simulink library "IO"  (R2024a)
settings: Solver=VariableStepAuto  StartTime=0.0  StopTime=10.0  RelTol=1e-3
values from neighbouring files (symbols this model uses):
  ADCBits = 12.0    [IO.sldd]
  Vref = 5.0    [IO.sldd]
undefined symbols (not defined in the file or in its folder): Bridge, dt, H, raptor_xcp_function
libraries: Raptor_lib x69, Utilities x20, Cooling x1
(part 3 of 3)

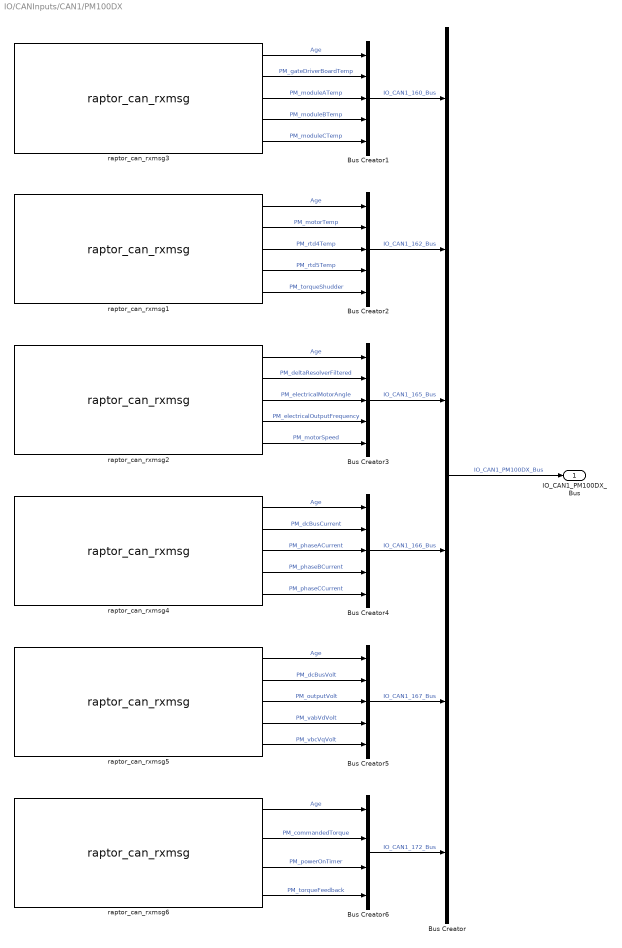
== system IO/CANInputs/CAN1/PM100DX ==
  Bus Creator : BusCreator  Inputs=6
  Bus Creator{1..5} (5 alike) : BusCreator  Inputs=5
  Bus Creator6 : BusCreator  Inputs=4
  raptor_can_rxmsg1 : Raptor_lib/CAN/raptor_can_rxmsg  canDefinition=struct('dbcFile', 'SR26_CAN1.dbc','message', 'PM_162','comment', '','signals', {{'PM_motorTemp','PM_rtd4Temp','PM_rtd5Temp','PM_torqueShudder'}},'enabled', [ 1 1 1 1;],'scaled', [ 1 1 1 1;],'canBus', '''CAN1''','messageID', [ 162;],'idMask', [ 536870911;],'payloadMask', [],'payloadValue', [],'period', [ 0;],'mailbox', '''''','queueSize', [ 1;],'label', [ 0;],'ver', [ 2;],'showID', [ 0;],'showRaw', [ 0;],'showRawMsg', [ 0;],'useStartVals', [ 0;],'extendedId', [ 0;],'showAge', [ 1;],'useSimFunc', [ 0;],'sim_func_name', '''''','fill', [ 0;],'editID', [ 0;],'signalOrder', [ 1;],'signalAscDes', [ 1;],'msgLength', [ 8;])  canBus='CAN1'  mailbox=''  payloadMask=[]  payloadValue=[]  idMask=hex2dec('1FFFFFFF')  queueSize=1  showID=0  label=0  fill=0  id=162  showRaw=0  showAge=1  signalOrder=1  signalInfo={{struct('Name', 'PM_torqueShudder','StartBit', [ 48;],'SignalSize', [ 16;],'ByteOrder', 'LittleEndian','ValueType', 'SIGNED','Class', 'int16','Signed', [ 1;],'Factor', [ 0.1;],'Offset', [ 0;],'Min', [ -3276.8;],'Max', [ 3276.7;],'Units', 'Nm','StartVal', [ 0;],'Comment', 'Shudder Compensation Value of Torque','Multiplexed', [ 0;],'Multiplexor', [ 0;],'MultiplexMode_Min', [],'MultiplexMode_Max', []),struct('Name', 'PM_motorTemp','StartBit', [ 32;],'SignalSize', [ 16;],'ByteOrder', 'LittleEndian','ValueType', 'SIGNED','Class', 'int16','Signed', [ 1;],'Factor', [ 0.1;],'Offset', [ 0;],'Min', [ -3276.8;],'Max', [ 3276.7;],'Units', 'degC','StartVal', [ 0;],'Comment', 'Motor Temperature Sensor','Multiplexed', [ 0;],'Multiplexor', [ 0;],'MultiplexMode_Min', [],'MultiplexMode_Max', []),struct('Name', 'PM_rtd5Temp','StartBit', [ 16;],'SignalSize', [ 16;],'ByteOrder', 'LittleEndian','ValueType', 'SIGNED','Class', 'int16','Signed', [ 1;],'Factor', [ 0.1;],'Offset', [ 0;],'Min', [ -3276.8;],'Max', [ 3276.7;],'Units', 'degC','StartVal', [ 0;],'Comment', 'RTD Input 5 (PT1000) Temperature (Gen 2 Only)','Multiplexed', [ 0;],'Multiplexor', [ 0;],'MultiplexMode_Min', [],'MultiplexMode_Max', []),struct('Name', 'PM_rtd4Temp','StartBit', [ 0;],'SignalSize', [ 16;],'ByteOrder', 'LittleEndian','ValueType', 'SIGNED','Class', 'int16','Signed', [ 1;],'Factor', [ 0.1;],'Offset', [ 0;],'Min', [ -3276.8;],'Max', [ 3276.7;],'Units', 'degC','StartVal', [ 0;],'Comment', 'RTD Input 4 (PT1000) Temperature (Gen 2 Only)','Multiplexed', [ 0;],'Multiplexor', [ 0;],'MultiplexMode_Min', [],'MultiplexMode_Max', [])}}  showRawMsg=0  useSimFunc=0  sim_func_name=''  useStartVals=0  extendedId=0
      settings: SourceProductName=Raptor
  raptor_can_rxmsg2 : Raptor_lib/CAN/raptor_can_rxmsg  canDefinition=struct('dbcFile', 'SR26_CAN1.dbc','message', 'PM_165','comment', '','signals', {{'PM_deltaResolverFiltered','PM_electricalMotorAngle','PM_electricalOutputFrequency','PM_motorSpeed'}},'enabled', [ 1 1 1 1;],'scaled', [ 1 1 1 1;],'canBus', '''CAN1''','messageID', [ 165;],'idMask', [ 536870911;],'payloadMask', [],'payloadValue', [],'period', [ 0;],'mailbox', '''''','queueSize', [ 1;],'label', [ 0;],'ver', [ 2;],'showID', [ 0;],'showRaw', [ 0;],'showRawMsg', [ 0;],'useStartVals', [ 0;],'extendedId', [ 0;],'showAge', [ 1;],'useSimFunc', [ 0;],'sim_func_name', '''''','fill', [ 0;],'editID', [ 0;],'signalOrder', [ 1;],'signalAscDes', [ 1;],'msgLength', [ 8;])  canBus='CAN1'  mailbox=''  payloadMask=[]  payloadValue=[]  idMask=hex2dec('1FFFFFFF')  queueSize=1  showID=0  label=0  fill=0  id=165  showRaw=0  showAge=1  signalOrder=1  signalInfo={{struct('Name', 'PM_deltaResolverFiltered','StartBit', [ 48;],'SignalSize', [ 16;],'ByteOrder', 'LittleEndian','ValueType', 'SIGNED','Class', 'int16','Signed', [ 1;],'Factor', [ 0.1;],'Offset', [ 0;],'Min', [ -3276.8;],'Max', [ 3276.7;],'Units', 'deg','StartVal', [ 0;],'Comment', 'Used in calibration of resolver angle adjustment','Multiplexed', [ 0;],'Multiplexor', [ 0;],'MultiplexMode_Min', [],'MultiplexMode_Max', []),struct('Name', 'PM_electricalOutputFrequency','StartBit', [ 32;],'SignalSize', [ 16;],'ByteOrder', 'LittleEndian','ValueType', 'SIGNED','Class', 'int16','Signed', [ 1;],'Factor', [ 0.1;],'Offset', [ 0;],'Min', [ -3276.8;],'Max', [ 3276.7;],'Units', 'Hz','StartVal', [ 0;],'Comment', 'The actual frequency of the inverter','Multiplexed', [ 0;],'Multiplexor', [ 0;],'MultiplexMode_Min', [],'MultiplexMode_Max', []),struct('Name', 'PM_motorSpeed','StartBit', [ 16;],'SignalSize', [ 16;],'ByteOrder', 'LittleEndian','ValueType', 'SIGNED','Class', 'int16','Signed', [ 1;],'Factor', [ 1;],'Offset', [ 0;],'Min', [ -32768;],'Max', [ 32767;],'Units', 'rpm','StartVal', [ 0;],'Comment', 'The measured speed of the motor','Multiplexed', [ 0;],'Multiplexor', [ 0;],'MultiplexMode_Min', [],'MultiplexMode_Max', []),struct('Name', 'PM_electricalMotorAngle','StartBit', [ 0;],'SignalSize', [ 16;],'ByteOrder', 'LittleEndian','ValueType', 'UNSIGNED','Class', 'uint16','Signed', [ 0;],'Factor', [ 0.1;],'Offset', [ 0;],'Min', [ 0;],'Max', [ 6553.5;],'Units', 'deg','StartVal', [ 0;],'Comment', 'The Electrical Angle of the motor as read by the encoder or resolver','Multiplexed', [ 0;],'Multiplexor', [ 0;],'MultiplexMode_Min', [],'MultiplexMode_Max', [])}}  showRawMsg=0  useSimFunc=0  sim_func_name=''  useStartVals=0  extendedId=0
      settings: SourceProductName=Raptor
  raptor_can_rxmsg3 : Raptor_lib/CAN/raptor_can_rxmsg  canDefinition=struct('dbcFile', 'SR26_CAN1.dbc','message', 'PM_160','comment', '','signals', {{'PM_gateDriverBoardTemp','PM_moduleATemp','PM_moduleBTemp','PM_moduleCTemp'}},'enabled', [ 1 1 1 1;],'scaled', [ 1 1 1 1;],'canBus', '''CAN1''','messageID', [ 160;],'idMask', [ 536870911;],'payloadMask', [],'payloadValue', [],'period', [ 0;],'mailbox', '''''','queueSize', [ 1;],'label', [ 0;],'ver', [ 2;],'showID', [ 0;],'showRaw', [ 0;],'showRawMsg', [ 0;],'useStartVals', [ 0;],'extendedId', [ 0;],'showAge', [ 1;],'useSimFunc', [ 0;],'sim_func_name', '''''','fill', [ 0;],'editID', [ 0;],'signalOrder', [ 1;],'signalAscDes', [ 1;],'msgLength', [ 8;])  canBus='CAN1'  mailbox=''  payloadMask=[]  payloadValue=[]  idMask=hex2dec('1FFFFFFF')  queueSize=1  showID=0  label=0  fill=0  id=160  showRaw=0  showAge=1  signalOrder=1  signalInfo={{struct('Name', 'PM_gateDriverBoardTemp','StartBit', [ 48;],'SignalSize', [ 16;],'ByteOrder', 'LittleEndian','ValueType', 'SIGNED','Class', 'int16','Signed', [ 1;],'Factor', [ 0.1;],'Offset', [ 0;],'Min', [ -3276.8;],'Max', [ 3276.7;],'Units', 'degC','StartVal', [ 0;],'Comment', 'Gate Driver Board Temperature','Multiplexed', [ 0;],'Multiplexor', [ 0;],'MultiplexMode_Min', [],'MultiplexMode_Max', []),struct('Name', 'PM_moduleCTemp','StartBit', [ 32;],'SignalSize', [ 16;],'ByteOrder', 'LittleEndian','ValueType', 'SIGNED','Class', 'int16','Signed', [ 1;],'Factor', [ 0.1;],'Offset', [ 0;],'Min', [ -3276.8;],'Max', [ 3276.7;],'Units', 'degC','StartVal', [ 0;],'Comment', 'IGBT Module C Temperature','Multiplexed', [ 0;],'Multiplexor', [ 0;],'MultiplexMode_Min', [],'MultiplexMode_Max', []),struct('Name', 'PM_moduleBTemp','StartBit', [ 16;],'SignalSize', [ 16;],'ByteOrder', 'LittleEndian','ValueType', 'SIGNED','Class', 'int16','Signed', [ 1;],'Factor', [ 0.1;],'Offset', [ 0;],'Min', [ -3276.8;],'Max', [ 3276.7;],'Units', 'degC','StartVal', [ 0;],'Comment', 'IGBT Module B Temperature','Multiplexed', [ 0;],'Multiplexor', [ 0;],'MultiplexMode_Min', [],'MultiplexMode_Max', []),struct('Name', 'PM_moduleATemp','StartBit', [ 0;],'SignalSize', [ 16;],'ByteOrder', 'LittleEndian','ValueType', 'SIGNED','Class', 'int16','Signed', [ 1;],'Factor', [ 0.1;],'Offset', [ 0;],'Min', [ -3276.8;],'Max', [ 3276.7;],'Units', 'degC','StartVal', [ 0;],'Comment', 'IGBT Module A Temperature','Multiplexed', [ 0;],'Multiplexor', [ 0;],'MultiplexMode_Min', [],'MultiplexMode_Max', [])}}  showRawMsg=0  useSimFunc=0  sim_func_name=''  useStartVals=0  extendedId=0
      settings: SourceProductName=Raptor
  raptor_can_rxmsg4 : Raptor_lib/CAN/raptor_can_rxmsg  canDefinition=struct('dbcFile', 'SR26_CAN1.dbc','message', 'PM_166','comment', '','signals', {{'PM_dcBusCurrent','PM_phaseACurrent','PM_phaseBCurrent','PM_phaseCCurrent'}},'enabled', [ 1 1 1 1;],'scaled', [ 1 1 1 1;],'canBus', '''CAN1''','messageID', [ 166;],'idMask', [ 536870911;],'payloadMask', [],'payloadValue', [],'period', [ 0;],'mailbox', '''''','queueSize', [ 1;],'label', [ 0;],'ver', [ 2;],'showID', [ 0;],'showRaw', [ 0;],'showRawMsg', [ 0;],'useStartVals', [ 0;],'extendedId', [ 0;],'showAge', [ 1;],'useSimFunc', [ 0;],'sim_func_name', '''''','fill', [ 0;],'editID', [ 0;],'signalOrder', [ 1;],'signalAscDes', [ 1;],'msgLength', [ 8;])  canBus='CAN1'  mailbox=''  payloadMask=[]  payloadValue=[]  idMask=hex2dec('1FFFFFFF')  queueSize=1  showID=0  label=0  fill=0  id=166  showRaw=0  showAge=1  signalOrder=1  signalInfo={{struct('Name', 'PM_dcBusCurrent','StartBit', [ 48;],'SignalSize', [ 16;],'ByteOrder', 'LittleEndian','ValueType', 'SIGNED','Class', 'int16','Signed', [ 1;],'Factor', [ 0.1;],'Offset', [ 0;],'Min', [ -3276.8;],'Max', [ 3276.7;],'Units', 'A','StartVal', [ 0;],'Comment', 'The calculated DC Bus Current','Multiplexed', [ 0;],'Multiplexor', [ 0;],'MultiplexMode_Min', [],'MultiplexMode_Max', []),struct('Name', 'PM_phaseCCurrent','StartBit', [ 32;],'SignalSize', [ 16;],'ByteOrder', 'LittleEndian','ValueType', 'SIGNED','Class', 'int16','Signed', [ 1;],'Factor', [ 0.1;],'Offset', [ 0;],'Min', [ -3276.8;],'Max', [ 3276.7;],'Units', 'A','StartVal', [ 0;],'Comment', 'The measured value of Phase C current','Multiplexed', [ 0;],'Multiplexor', [ 0;],'MultiplexMode_Min', [],'MultiplexMode_Max', []),struct('Name', 'PM_phaseBCurrent','StartBit', [ 16;],'SignalSize', [ 16;],'ByteOrder', 'LittleEndian','ValueType', 'SIGNED','Class', 'int16','Signed', [ 1;],'Factor', [ 0.1;],'Offset', [ 0;],'Min', [ -3276.8;],'Max', [ 3276.7;],'Units', 'A','StartVal', [ 0;],'Comment', 'The measured value of Phase B current','Multiplexed', [ 0;],'Multiplexor', [ 0;],'MultiplexMode_Min', [],'MultiplexMode_Max', []),struct('Name', 'PM_phaseACurrent','StartBit', [ 0;],'SignalSize', [ 16;],'ByteOrder', 'LittleEndian','ValueType', 'SIGNED','Class', 'int16','Signed', [ 1;],'Factor', [ 0.1;],'Offset', [ 0;],'Min', [ -3276.8;],'Max', [ 3276.7;],'Units', 'A','StartVal', [ 0;],'Comment', 'The measured value of Phase A current','Multiplexed', [ 0;],'Multiplexor', [ 0;],'MultiplexMode_Min', [],'MultiplexMode_Max', [])}}  showRawMsg=0  useSimFunc=0  sim_func_name=''  useStartVals=0  extendedId=0
      settings: SourceProductName=Raptor
  raptor_can_rxmsg5 : Raptor_lib/CAN/raptor_can_rxmsg  canDefinition=struct('dbcFile', 'SR26_CAN1.dbc','message', 'PM_167','comment', '','signals', {{'PM_dcBusVolt','PM_outputVolt','PM_vabVdVolt','PM_vbcVqVolt'}},'enabled', [ 1 1 1 1;],'scaled', [ 1 1 1 1;],'canBus', '''CAN1''','messageID', [ 167;],'idMask', [ 536870911;],'payloadMask', [],'payloadValue', [],'period', [ 0;],'mailbox', '''''','queueSize', [ 1;],'label', [ 0;],'ver', [ 2;],'showID', [ 0;],'showRaw', [ 0;],'showRawMsg', [ 0;],'useStartVals', [ 0;],'extendedId', [ 0;],'showAge', [ 1;],'useSimFunc', [ 0;],'sim_func_name', '''''','fill', [ 0;],'editID', [ 0;],'signalOrder', [ 1;],'signalAscDes', [ 1;],'msgLength', [ 8;])  canBus='CAN1'  mailbox=''  payloadMask=[]  payloadValue=[]  idMask=hex2dec('1FFFFFFF')  queueSize=1  showID=0  label=0  fill=0  id=167  showRaw=0  showAge=1  signalOrder=1  signalInfo={{struct('Name', 'PM_vbcVqVolt','StartBit', [ 48;],'SignalSize', [ 16;],'ByteOrder', 'LittleEndian','ValueType', 'SIGNED','Class', 'int16','Signed', [ 1;],'Factor', [ 0.1;],'Offset', [ 0;],'Min', [ -3276.8;],'Max', [ 3276.7;],'Units', 'V','StartVal', [ 0;],'Comment', 'Measured value of the voltage between Phase B and Phase C','Multiplexed', [ 0;],'Multiplexor', [ 0;],'MultiplexMode_Min', [],'MultiplexMode_Max', []),struct('Name', 'PM_vabVdVolt','StartBit', [ 32;],'SignalSize', [ 16;],'ByteOrder', 'LittleEndian','ValueType', 'SIGNED','Class', 'int16','Signed', [ 1;],'Factor', [ 0.1;],'Offset', [ 0;],'Min', [ -3276.8;],'Max', [ 3276.7;],'Units', 'V','StartVal', [ 0;],'Comment', 'Measured value of the voltage between Phase A and Phase B','Multiplexed', [ 0;],'Multiplexor', [ 0;],'MultiplexMode_Min', [],'MultiplexMode_Max', []),struct('Name', 'PM_outputVolt','StartBit', [ 16;],'SignalSize', [ 16;],'ByteOrder', 'LittleEndian','ValueType', 'SIGNED','Class', 'int16','Signed', [ 1;],'Factor', [ 0.1;],'Offset', [ 0;],'Min', [ -3276.8;],'Max', [ 3276.7;],'Units', 'V','StartVal', [ 0;],'Comment', 'The calculated value of the output voltage, in peak line-neutral volts','Multiplexed', [ 0;],'Multiplexor', [ 0;],'MultiplexMode_Min', [],'MultiplexMode_Max', []),struct('Name', 'PM_dcBusVolt','StartBit', [ 0;],'SignalSize', [ 16;],'ByteOrder', 'LittleEndian','ValueType', 'SIGNED','Class', 'int16','Signed', [ 1;],'Factor', [ 0.1;],'Offset', [ 0;],'Min', [ -3276.8;],'Max', [ 3276.7;],'Units', 'V','StartVal', [ 0;],'Comment', 'The actual measured value of the DC bus voltage','Multiplexed', [ 0;],'Multiplexor', [ 0;],'MultiplexMode_Min', [],'MultiplexMode_Max', [])}}  showRawMsg=0  useSimFunc=0  sim_func_name=''  useStartVals=0  extendedId=0
      settings: SourceProductName=Raptor
  raptor_can_rxmsg6 : Raptor_lib/CAN/raptor_can_rxmsg  canDefinition=struct('dbcFile', 'SR26_CAN1.dbc','message', 'PM_172','comment', '','signals', {{'PM_commandedTorque','PM_powerOnTimer','PM_torqueFeedback'}},'enabled', [ 1 1 1;],'scaled', [ 1 1 1;],'canBus', '''CAN1''','messageID', [ 172;],'idMask', [ 536870911;],'payloadMask', [],'payloadValue', [],'period', [ 0;],'mailbox', '''''','queueSize', [ 1;],'label', [ 0;],'ver', [ 2;],'showID', [ 0;],'showRaw', [ 0;],'showRawMsg', [ 0;],'useStartVals', [ 0;],'extendedId', [ 0;],'showAge', [ 1;],'useSimFunc', [ 0;],'sim_func_name', '''''','fill', [ 0;],'editID', [ 0;],'signalOrder', [ 1;],'signalAscDes', [ 1;],'msgLength', [ 8;])  canBus='CAN1'  mailbox=''  payloadMask=[]  payloadValue=[]  idMask=hex2dec('1FFFFFFF')  queueSize=1  showID=0  label=0  fill=0  id=172  showRaw=0  showAge=1  signalOrder=1  signalInfo={{struct('Name', 'PM_powerOnTimer','StartBit', [ 32;],'SignalSize', [ 32;],'ByteOrder', 'LittleEndian','ValueType', 'UNSIGNED','Class', 'uint32','Signed', [ 0;],'Factor', [ 0.003;],'Offset', [ 0;],'Min', [ 0;],'Max', [ 12884800;],'Units', 'sec','StartVal', [ 0;],'Comment', 'Updated every 3 msec. This will roll over in approximately 150 days!','Multiplexed', [ 0;],'Multiplexor', [ 0;],'MultiplexMode_Min', [],'MultiplexMode_Max', []),struct('Name', 'PM_torqueFeedback','StartBit', [ 16;],'SignalSize', [ 16;],'ByteOrder', 'LittleEndian','ValueType', 'SIGNED','Class', 'int16','Signed', [ 1;],'Factor', [ 0.1;],'Offset', [ 0;],'Min', [ -3276.8;],'Max', [ 3276.7;],'Units', 'Nm','StartVal', [ 0;],'Comment', 'Estimated motor torque feedback','Multiplexed', [ 0;],'Multiplexor', [ 0;],'MultiplexMode_Min', [],'MultiplexMode_Max', []),struct('Name', 'PM_commandedTorque','StartBit', [ 0;],'SignalSize', [ 16;],'ByteOrder', 'LittleEndian','ValueType', 'SIGNED','Class', 'int16','Signed', [ 1;],'Factor', [ 0.1;],'Offset', [ 0;],'Min', [ -3276.8;],'Max', [ 3276.7;],'Units', 'Nm','StartVal', [ 0;],'Comment', 'The commanded torque','Multiplexed', [ 0;],'Multiplexor', [ 0;],'MultiplexMode_Min', [],'MultiplexMode_Max', [])}}  showRawMsg=0  useSimFunc=0  sim_func_name=''  useStartVals=0  extendedId=0
      settings: SourceProductName=Raptor
  IO_CAN1_PM100DX_Bus : Outport
  wires:
  Bus Creator3/1 -> Bus Creator/3  "IO_CAN1_165_Bus"
  Bus Creator4/1 -> Bus Creator/4  "IO_CAN1_166_Bus"
  raptor_can_rxmsg6/4 -> Bus Creator6/4  "PM_torqueFeedback"
  raptor_can_rxmsg6/1 -> Bus Creator6/1  "Age"
  raptor_can_rxmsg6/2 -> Bus Creator6/2  "PM_commandedTorque"
  raptor_can_rxmsg6/3 -> Bus Creator6/3  "PM_powerOnTimer"
  Bus Creator6/1 -> Bus Creator/6  "IO_CAN1_172_Bus"
  Bus Creator5/1 -> Bus Creator/5  "IO_CAN1_167_Bus"
  raptor_can_rxmsg5/5 -> Bus Creator5/5  "PM_vbcVqVolt"
  raptor_can_rxmsg5/4 -> Bus Creator5/4  "PM_vabVdVolt"
  raptor_can_rxmsg5/3 -> Bus Creator5/3  "PM_outputVolt"
  raptor_can_rxmsg5/2 -> Bus Creator5/2  "PM_dcBusVolt"
  raptor_can_rxmsg5/1 -> Bus Creator5/1  "Age"
  raptor_can_rxmsg4/1 -> Bus Creator4/1  "Age"
  raptor_can_rxmsg4/2 -> Bus Creator4/2  "PM_dcBusCurrent"
  raptor_can_rxmsg4/3 -> Bus Creator4/3  "PM_phaseACurrent"
  raptor_can_rxmsg4/4 -> Bus Creator4/4  "PM_phaseBCurrent"
  raptor_can_rxmsg4/5 -> Bus Creator4/5  "PM_phaseCCurrent"
  raptor_can_rxmsg2/5 -> Bus Creator3/5  "PM_motorSpeed"
  raptor_can_rxmsg2/4 -> Bus Creator3/4  "PM_electricalOutputFrequency"
  raptor_can_rxmsg2/3 -> Bus Creator3/3  "PM_electricalMotorAngle"
  raptor_can_rxmsg2/2 -> Bus Creator3/2  "PM_deltaResolverFiltered"
  raptor_can_rxmsg2/1 -> Bus Creator3/1  "Age"
  raptor_can_rxmsg3/5 -> Bus Creator1/5  "PM_moduleCTemp"
  raptor_can_rxmsg3/4 -> Bus Creator1/4  "PM_moduleBTemp"
  raptor_can_rxmsg3/3 -> Bus Creator1/3  "PM_moduleATemp"
  raptor_can_rxmsg3/2 -> Bus Creator1/2  "PM_gateDriverBoardTemp"
  Bus Creator1/1 -> Bus Creator/1  "IO_CAN1_160_Bus"
  raptor_can_rxmsg3/1 -> Bus Creator1/1  "Age"
  Bus Creator/1 -> IO_CAN1_PM100DX_Bus/1  "IO_CAN1_PM100DX_Bus"
  raptor_can_rxmsg1/1 -> Bus Creator2/1  "Age"
  raptor_can_rxmsg1/2 -> Bus Creator2/2  "PM_motorTemp"
  raptor_can_rxmsg1/3 -> Bus Creator2/3  "PM_rtd4Temp"
  raptor_can_rxmsg1/4 -> Bus Creator2/4  "PM_rtd5Temp"
  raptor_can_rxmsg1/5 -> Bus Creator2/5  "PM_torqueShudder"
  Bus Creator2/1 -> Bus Creator/2  "IO_CAN1_162_Bus"

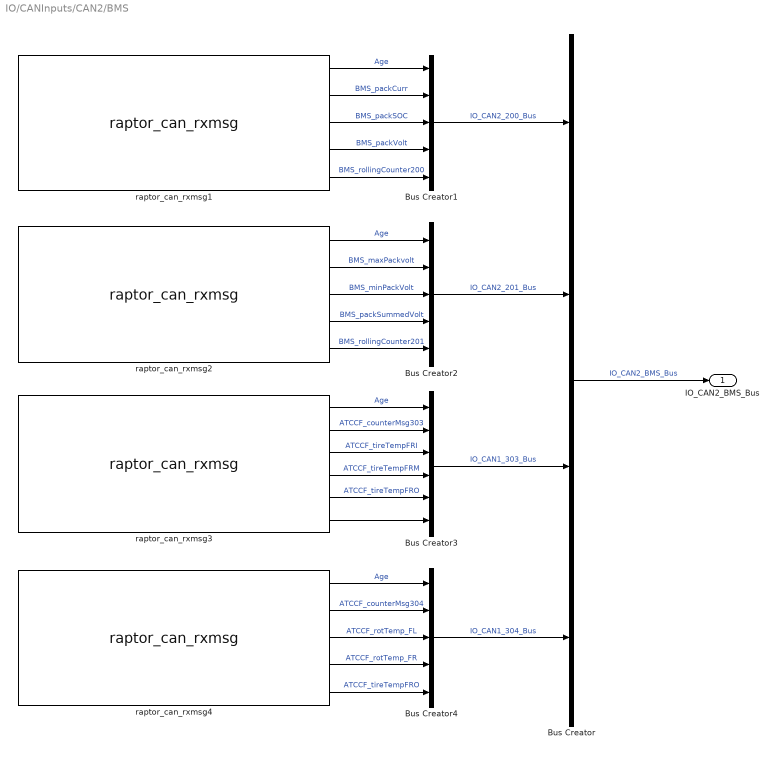
== system IO/CANInputs/CAN2/BMS ==
  Bus Creator : BusCreator  Inputs=4
  Bus Creator1 : BusCreator  Inputs=5
  Bus Creator2 : BusCreator  Inputs=5
  Bus Creator3 : BusCreator  Inputs=6
  Bus Creator4 : BusCreator  Inputs=5
  raptor_can_rxmsg1 : Raptor_lib/CAN/raptor_can_rxmsg  canDefinition=struct('dbcFile', 'SR26_CAN2.dbc','message', 'BMS_200','comment', '','signals', {{'BMS_packCurr','BMS_packSOC','BMS_packVolt','BMS_rollingCounter200'}},'enabled', [ 1 1 1 1;],'scaled', [ 1 1 1 1;],'canBus', '''CAN2''','messageID', [ 200;],'idMask', [ 536870911;],'payloadMask', [],'payloadValue', [],'period', [ 0;],'mailbox', '''''','queueSize', [ 1;],'label', [ 0;],'ver', [ 2;],'showID', [ 0;],'showRaw', [ 0;],'showRawMsg', [ 0;],'useStartVals', [ 0;],'extendedId', [ 0;],'showAge', [ 1;],'useSimFunc', [ 0;],'sim_func_name', '''''','fill', [ 0;],'editID', [ 0;],'signalOrder', [ 1;],'signalAscDes', [ 1;],'msgLength', [ 8;])  canBus='CAN2'  mailbox=''  payloadMask=[]  payloadValue=[]  idMask=hex2dec('1FFFFFFF')  queueSize=1  showID=0  label=0  fill=0  id=200  showRaw=0  showAge=1  signalOrder=1  signalInfo={{struct('Name', 'BMS_packSOC','StartBit', [ 48;],'SignalSize', [ 8;],'ByteOrder', 'LittleEndian','ValueType', 'SIGNED','Class', 'int8','Signed', [ 1;],'Factor', [ 0.5;],'Offset', [ 0;],'Min', [ 0;],'Max', [ 100;],'Units', '%','StartVal', [ 0;],'Comment', 'This is the pack State of Charge','Multiplexed', [ 0;],'Multiplexor', [ 0;],'MultiplexMode_Min', [],'MultiplexMode_Max', []),struct('Name', 'BMS_packVolt','StartBit', [ 32;],'SignalSize', [ 16;],'ByteOrder', 'LittleEndian','ValueType', 'SIGNED','Class', 'int16','Signed', [ 1;],'Factor', [ 0.1;],'Offset', [ 0;],'Min', [ -3276.8;],'Max', [ 3276.7;],'Units', 'V','StartVal', [ 0;],'Comment', 'This is the instantaneous total pack voltage value','Multiplexed', [ 0;],'Multiplexor', [ 0;],'MultiplexMode_Min', [],'MultiplexMode_Max', []),struct('Name', 'BMS_packCurr','StartBit', [ 16;],'SignalSize', [ 16;],'ByteOrder', 'LittleEndian','ValueType', 'SIGNED','Class', 'int16','Signed', [ 1;],'Factor', [ 0.1;],'Offset', [ 0;],'Min', [ -3276.8;],'Max', [ 3276.7;],'Units', 'A','StartVal', [ 0;],'Comment', 'This is the current pack amperage value for the battery pack. This will report a constant 0 if no current sensor is selected','Multiplexed', [ 0;],'Multiplexor', [ 0;],'MultiplexMode_Min', [],'MultiplexMode_Max', []),struct('Name', 'BMS_rollingCounter200','StartBit', [ 0;],'SignalSize', [ 8;],'ByteOrder', 'LittleEndian','ValueType', 'UNSIGNED','Class', 'uint8','Signed', [ 0;],'Factor', [ 1;],'Offset', [ 0;],'Min', [ 0;],'Max', [ 255;],'Units', '','StartVal', [ 0;],'Comment', 'Increments once every 100ms (max value is 255 and rolls over). Can be used to ensure data is updating','Multiplexed', [ 0;],'Multiplexor', [ 0;],'MultiplexMode_Min', [],'MultiplexMode_Max', [])}}  showRawMsg=0  useSimFunc=0  sim_func_name=''  useStartVals=0  extendedId=0
      settings: SourceProductName=Raptor
  raptor_can_rxmsg2 : Raptor_lib/CAN/raptor_can_rxmsg  canDefinition=struct('dbcFile', 'SR26_CAN2.dbc','message', 'BMS_201','comment', '','signals', {{'BMS_maxPackVolt','BMS_minPackVolt','BMS_packSummedVolt','BMS_rollingCounter201'}},'enabled', [ 1 1 1 1;],'scaled', [ 1 1 1 1;],'canBus', '''CAN2''','messageID', [ 201;],'idMask', [ 536870911;],'payloadMask', [],'payloadValue', [],'period', [ 0;],'mailbox', '''''','queueSize', [ 1;],'label', [ 0;],'ver', [ 2;],'showID', [ 0;],'showRaw', [ 0;],'showRawMsg', [ 0;],'useStartVals', [ 0;],'extendedId', [ 0;],'showAge', [ 1;],'useSimFunc', [ 0;],'sim_func_name', '''''','fill', [ 0;],'editID', [ 0;],'signalOrder', [ 1;],'signalAscDes', [ 1;],'msgLength', [ 8;])  canBus='CAN2'  mailbox=''  payloadMask=[]  payloadValue=[]  idMask=hex2dec('1FFFFFFF')  queueSize=1  showID=0  label=0  fill=0  id=201  showRaw=0  showAge=1  signalOrder=1  signalInfo={{struct('Name', 'BMS_minPackVolt','StartBit', [ 48;],'SignalSize', [ 16;],'ByteOrder', 'LittleEndian','ValueType', 'SIGNED','Class', 'int16','Signed', [ 1;],'Factor', [ 0.1;],'Offset', [ 0;],'Min', [ -3276.8;],'Max', [ 3276.7;],'Units', 'V','StartVal', [ 0;],'Comment', 'This value is the mainimum pack voltage that the BMS is using to limit how low the pack voltage is allowed to be pulled down to','Multiplexed', [ 0;],'Multiplexor', [ 0;],'MultiplexMode_Min', [],'MultiplexMode_Max', []),struct('Name', 'BMS_maxPackVolt','StartBit', [ 32;],'SignalSize', [ 16;],'ByteOrder', 'LittleEndian','ValueType', 'SIGNED','Class', 'int16','Signed', [ 1;],'Factor', [ 0.1;],'Offset', [ 0;],'Min', [ -3276.8;],'Max', [ 3276.7;],'Units', 'V','StartVal', [ 0;],'Comment', 'This value is the maximum pack voltage that the BMS is using to limit how high the pack voltage can be. This can be useful for communicating with chargers or charging stations expecting a maximum pack voltage value they are able to charge up to','Multiplexed', [ 0;],'Multiplexor', [ 0;],'MultiplexMode_Min', [],'MultiplexMode_Max', []),struct('Name', 'BMS_packSummedVolt','StartBit', [ 16;],'SignalSize', [ 16;],'ByteOrder', 'LittleEndian','ValueType', 'SIGNED','Class', 'int16','Signed', [ 1;],'Factor', [ 0.01;],'Offset', [ 0;],'Min', [ -327.68;],'Max', [ 327.67;],'Units', 'V','StartVal', [ 0;],'Comment', 'This value is the sum of all the cells being monitored by the BMS and represents the overall pack voltage. It is essentially identical to the Pack Voltage value, except that it is reported wit ha higher resolution (0.01V versus 0.1V)','Multiplexed', [ 0;],'Multiplexor', [ 0;],'MultiplexMode_Min', [],'MultiplexMode_Max', []),struct('Name', 'BMS_rollingCounter201','StartBit', [ 0;],'SignalSize', [ 8;],'ByteOrder', 'LittleEndian','ValueType', 'UNSIGNED','Class', 'uint8','Signed', [ 0;],'Factor', [ 1;],'Offset', [ 0;],'Min', [ 0;],'Max', [ 255;],'Units', '','StartVal', [ 0;],'Comment', 'Increments once every 100ms (max value is 255 and rolls over). Can be used to ensure data is updating','Multiplexed', [ 0;],'Multiplexor', [ 0;],'MultiplexMode_Min', [],'MultiplexMode_Max', [])}}  showRawMsg=0  useSimFunc=0  sim_func_name=''  useStartVals=0  extendedId=0
      settings: SourceProductName=Raptor
  raptor_can_rxmsg3 : Raptor_lib/CAN/raptor_can_rxmsg  canDefinition=struct('dbcFile', 'SR26_CAN2.dbc','message', 'BMS_202','comment', '','signals', {{'BMS_packAmphours','BMS_packDOD','BMS_packResistance','BMS_packSOH','BMS_rollingCounter202'}},'enabled', [ 1 1 1 1 1;],'scaled', [ 1 1 1 1 1;],'canBus', '''CAN2''','messageID', [ 202;],'idMask', [ 536870911;],'payloadMask', [],'payloadValue', [],'period', [ 0;],'mailbox', '''''','queueSize', [ 1;],'label', [ 0;],'ver', [ 2;],'showID', [ 0;],'showRaw', [ 0;],'showRawMsg', [ 0;],'useStartVals', [ 0;],'extendedId', [ 0;],'showAge', [ 1;],'useSimFunc', [ 0;],'sim_func_name', '''''','fill', [ 0;],'editID', [ 0;],'signalOrder', [ 1;],'signalAscDes', [ 1;],'msgLength', [ 8;])  canBus='CAN2'  mailbox=''  payloadMask=[]  payloadValue=[]  idMask=hex2dec('1FFFFFFF')  queueSize=1  showID=0  label=0  fill=0  id=202  showRaw=0  showAge=1  signalOrder=1  signalInfo={{struct('Name', 'BMS_packResistance','StartBit', [ 48;],'SignalSize', [ 16;],'ByteOrder', 'LittleEndian','ValueType', 'SIGNED','Class', 'int16','Signed', [ 1;],'Factor', [ 1;],'Offset', [ 0;],'Min', [ -32768;],'Max', [ 32767;],'Units', 'mOhm','StartVal', [ 0;],'Comment', 'This is the combined measured internal resistance for the entire battery pack','Multiplexed', [ 0;],'Multiplexor', [ 0;],'MultiplexMode_Min', [],'MultiplexMode_Max', []),struct('Name', 'BMS_packAmphours','StartBit', [ 32;],'SignalSize', [ 16;],'ByteOrder', 'LittleEndian','ValueType', 'SIGNED','Class', 'int16','Signed', [ 1;],'Factor', [ 0.1;],'Offset', [ 0;],'Min', [ -3276.8;],'Max', [ 3276.7;],'Units', 'Ahr','StartVal', [ 0;],'Comment', 'This is the calculated number of amphours remaining in the battery pack. This is used in part to calculate State of Charge','Multiplexed', [ 0;],'Multiplexor', [ 0;],'MultiplexMode_Min', [],'MultiplexMode_Max', []),struct('Name', 'BMS_packSOH','StartBit', [ 16;],'SignalSize', [ 8;],'ByteOrder', 'LittleEndian','ValueType', 'SIGNED','Class', 'int8','Signed', [ 1;],'Factor', [ 1;],'Offset', [ 0;],'Min', [ 0;],'Max', [ 100;],'Units', '%','StartVal', [ 0;],'Comment', 'This is the total state of health for the battery pack','Multiplexed', [ 0;],'Multiplexor', [ 0;],'MultiplexMode_Min', [],'MultiplexMode_Max', []),struct('Name', 'BMS_packDOD','StartBit', [ 8;],'SignalSize', [ 8;],'ByteOrder', 'LittleEndian','ValueType', 'SIGNED','Class', 'int8','Signed', [ 1;],'Factor', [ 0.5;],'Offset', [ 0;],'Min', [ 0;],'Max', [ 100;],'Units', '%','StartVal', [ 0;],'Comment', 'This value represents the total pack depth of discharge (that is, the total percent of the battery that has been discharged to this point). This value does not account for any Drift','Multiplexed', [ 0;],'Multiplexor', [ 0;],'MultiplexMode_Min', [],'MultiplexMode_Max', []),struct('Name', 'BMS_rollingCounter202','StartBit', [ 0;],'SignalSize', [ 8;],'ByteOrder', 'LittleEndian','ValueType', 'UNSIGNED','Class', 'uint8','Signed', [ 0;],'Factor', [ 1;],'Offset', [ 0;],'Min', [ 0;],'Max', [ 255;],'Units', '','StartVal', [ 0;],'Comment', 'Increments once every 100ms (max value is 255 and rolls over). Can be used to ensure data is updating','Multiplexed', [ 0;],'Multiplexor', [ 0;],'MultiplexMode_Min', [],'MultiplexMode_Max', [])}}  showRawMsg=0  useSimFunc=0  sim_func_name=''  useStartVals=0  extendedId=0
      settings: SourceProductName=Raptor
  raptor_can_rxmsg4 : Raptor_lib/CAN/raptor_can_rxmsg  canDefinition=struct('dbcFile', 'SR26_CAN2.dbc','message', 'BMS_201','comment', '','signals', {{'BMS_maxPackVolt','BMS_minPackVolt','BMS_packSummedVolt','BMS_rollingCounter201'}},'enabled', [ 1 1 1 1;],'scaled', [ 1 1 1 1;],'canBus', '''CAN2''','messageID', [ 201;],'idMask', [ 536870911;],'payloadMask', [],'payloadValue', [],'period', [ 0;],'mailbox', '''''','queueSize', [ 1;],'label', [ 0;],'ver', [ 2;],'showID', [ 0;],'showRaw', [ 0;],'showRawMsg', [ 0;],'useStartVals', [ 0;],'extendedId', [ 0;],'showAge', [ 1;],'useSimFunc', [ 0;],'sim_func_name', '''''','fill', [ 0;],'editID', [ 0;],'signalOrder', [ 1;],'signalAscDes', [ 1;],'msgLength', [ 8;])  canBus='CAN2'  mailbox=''  payloadMask=[]  payloadValue=[]  idMask=hex2dec('1FFFFFFF')  queueSize=1  showID=0  label=0  fill=0  id=201  showRaw=0  showAge=1  signalOrder=1  signalInfo={{struct('Name', 'BMS_minPackVolt','StartBit', [ 48;],'SignalSize', [ 16;],'ByteOrder', 'LittleEndian','ValueType', 'SIGNED','Class', 'int16','Signed', [ 1;],'Factor', [ 0.1;],'Offset', [ 0;],'Min', [ -3276.8;],'Max', [ 3276.7;],'Units', 'V','StartVal', [ 0;],'Comment', 'This value is the mainimum pack voltage that the BMS is using to limit how low the pack voltage is allowed to be pulled down to','Multiplexed', [ 0;],'Multiplexor', [ 0;],'MultiplexMode_Min', [],'MultiplexMode_Max', []),struct('Name', 'BMS_maxPackVolt','StartBit', [ 32;],'SignalSize', [ 16;],'ByteOrder', 'LittleEndian','ValueType', 'SIGNED','Class', 'int16','Signed', [ 1;],'Factor', [ 0.1;],'Offset', [ 0;],'Min', [ -3276.8;],'Max', [ 3276.7;],'Units', 'V','StartVal', [ 0;],'Comment', 'This value is the maximum pack voltage that the BMS is using to limit how high the pack voltage can be. This can be useful for communicating with chargers or charging stations expecting a maximum pack voltage value they are able to charge up to','Multiplexed', [ 0;],'Multiplexor', [ 0;],'MultiplexMode_Min', [],'MultiplexMode_Max', []),struct('Name', 'BMS_packSummedVolt','StartBit', [ 16;],'SignalSize', [ 16;],'ByteOrder', 'LittleEndian','ValueType', 'SIGNED','Class', 'int16','Signed', [ 1;],'Factor', [ 0.01;],'Offset', [ 0;],'Min', [ -327.68;],'Max', [ 327.67;],'Units', 'V','StartVal', [ 0;],'Comment', 'This value is the sum of all the cells being monitored by the BMS and represents the overall pack voltage. It is essentially identical to the Pack Voltage value, except that it is reported wit ha higher resolution (0.01V versus 0.1V)','Multiplexed', [ 0;],'Multiplexor', [ 0;],'MultiplexMode_Min', [],'MultiplexMode_Max', []),struct('Name', 'BMS_rollingCounter201','StartBit', [ 0;],'SignalSize', [ 8;],'ByteOrder', 'LittleEndian','ValueType', 'UNSIGNED','Class', 'uint8','Signed', [ 0;],'Factor', [ 1;],'Offset', [ 0;],'Min', [ 0;],'Max', [ 255;],'Units', '','StartVal', [ 0;],'Comment', 'Increments once every 100ms (max value is 255 and rolls over). Can be used to ensure data is updating','Multiplexed', [ 0;],'Multiplexor', [ 0;],'MultiplexMode_Min', [],'MultiplexMode_Max', [])}}  showRawMsg=0  useSimFunc=0  sim_func_name=''  useStartVals=0  extendedId=0
      settings: SourceProductName=Raptor
  IO_CAN2_BMS_Bus : Outport
  wires:
  raptor_can_rxmsg3/6 -> Bus Creator3/6
  raptor_can_rxmsg4/5 -> Bus Creator4/5  "ATCCF_tireTempFRO"
  raptor_can_rxmsg1/5 -> Bus Creator1/5  "BMS_rollingCounter200"
  Bus Creator1/1 -> Bus Creator/1  "IO_CAN2_200_Bus"
  raptor_can_rxmsg1/4 -> Bus Creator1/4  "BMS_packVolt"
  raptor_can_rxmsg1/3 -> Bus Creator1/3  "BMS_packSOC"
  raptor_can_rxmsg1/2 -> Bus Creator1/2  "BMS_packCurr"
  raptor_can_rxmsg1/1 -> Bus Creator1/1  "Age"
  raptor_can_rxmsg2/1 -> Bus Creator2/1  "Age"
  raptor_can_rxmsg2/2 -> Bus Creator2/2  "BMS_maxPackvolt"
  raptor_can_rxmsg2/3 -> Bus Creator2/3  "BMS_minPackVolt"
  raptor_can_rxmsg2/4 -> Bus Creator2/4  "BMS_packSummedVolt"
  Bus Creator2/1 -> Bus Creator/2  "IO_CAN2_201_Bus"
  raptor_can_rxmsg2/5 -> Bus Creator2/5  "BMS_rollingCounter201"
  raptor_can_rxmsg3/5 -> Bus Creator3/5  "ATCCF_tireTempFRO"
  Bus Creator3/1 -> Bus Creator/3  "IO_CAN1_303_Bus"
  raptor_can_rxmsg3/4 -> Bus Creator3/4  "ATCCF_tireTempFRM"
  raptor_can_rxmsg3/3 -> Bus Creator3/3  "ATCCF_tireTempFRI"
  raptor_can_rxmsg3/2 -> Bus Creator3/2  "ATCCF_counterMsg303"
  raptor_can_rxmsg3/1 -> Bus Creator3/1  "Age"
  raptor_can_rxmsg4/1 -> Bus Creator4/1  "Age"
  raptor_can_rxmsg4/2 -> Bus Creator4/2  "ATCCF_counterMsg304"
  raptor_can_rxmsg4/3 -> Bus Creator4/3  "ATCCF_rotTemp_FL"
  raptor_can_rxmsg4/4 -> Bus Creator4/4  "ATCCF_rotTemp_FR"
  Bus Creator4/1 -> Bus Creator/4  "IO_CAN1_304_Bus"
  Bus Creator/1 -> IO_CAN2_BMS_Bus/1  "IO_CAN2_BMS_Bus"

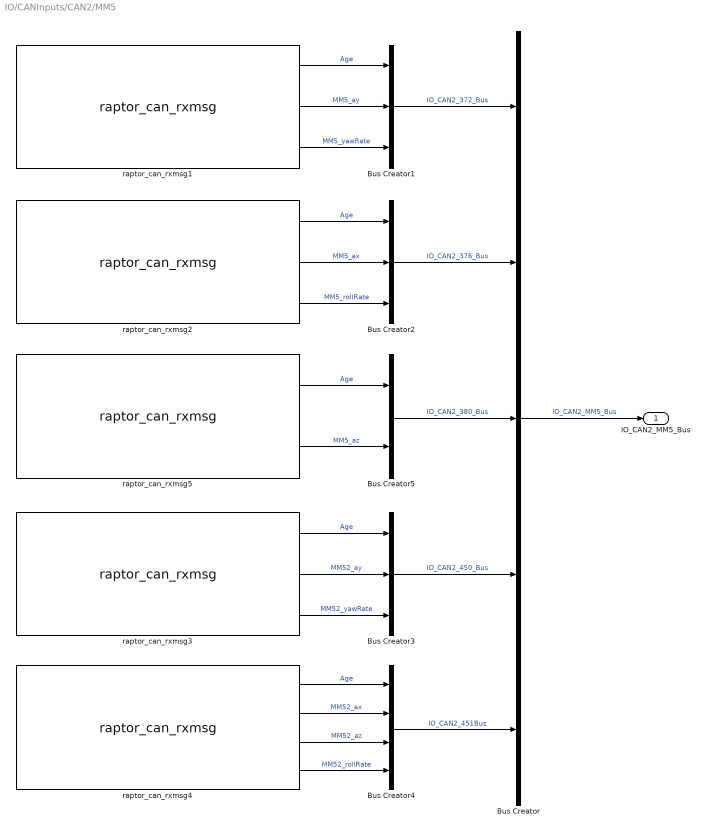
== system IO/CANInputs/CAN2/MM5 ==
  Bus Creator : BusCreator  Inputs=5
  Bus Creator1 : BusCreator  Inputs=3
  Bus Creator2 : BusCreator  Inputs=3
  Bus Creator3 : BusCreator  Inputs=3
  Bus Creator4 : BusCreator  Inputs=4
  Bus Creator5 : BusCreator  Inputs=2
  raptor_can_rxmsg1 : Raptor_lib/CAN/raptor_can_rxmsg  canDefinition=struct('dbcFile', 'SR26_CAN2.dbc','message', 'MM5_372','comment', '','signals', {{'MM5_ay','MM5_yawRate'}},'enabled', [ 1 1;],'scaled', [ 1 1;],'canBus', '''CAN2''','messageID', [ 372;],'idMask', [ 536870911;],'payloadMask', [],'payloadValue', [],'period', [ 0;],'mailbox', '''''','queueSize', [ 1;],'label', [ 0;],'ver', [ 2;],'showID', [ 0;],'showRaw', [ 0;],'showRawMsg', [ 0;],'useStartVals', [ 0;],'extendedId', [ 0;],'showAge', [ 1;],'useSimFunc', [ 0;],'sim_func_name', '''''','fill', [ 0;],'editID', [ 0;],'signalOrder', [ 1;],'signalAscDes', [ 1;],'msgLength', [ 8;])  canBus='CAN2'  mailbox=''  payloadMask=[]  payloadValue=[]  idMask=hex2dec('1FFFFFFF')  queueSize=1  showID=0  label=0  fill=0  id=372  showRaw=0  showAge=1  signalOrder=1  signalInfo={{struct('Name', 'MM5_ay','StartBit', [ 32;],'SignalSize', [ 16;],'ByteOrder', 'LittleEndian','ValueType', 'UNSIGNED','Class', 'uint16','Signed', [ 0;],'Factor', [ 0.0001274;],'Offset', [ -4.1746;],'Min', [ 0;],'Max', [ 0;],'Units', 'g','StartVal', [ 0;],'Comment', 'Acceleration Y Axis','Multiplexed', [ 0;],'Multiplexor', [ 0;],'MultiplexMode_Min', [],'MultiplexMode_Max', []),struct('Name', 'MM5_yawRate','StartBit', [ 0;],'SignalSize', [ 16;],'ByteOrder', 'LittleEndian','ValueType', 'UNSIGNED','Class', 'uint16','Signed', [ 0;],'Factor', [ 0.005;],'Offset', [ -163.9;],'Min', [ 0;],'Max', [ 0;],'Units', 'deg/sec','StartVal', [ 0;],'Comment', 'Yaw Rate','Multiplexed', [ 0;],'Multiplexor', [ 0;],'MultiplexMode_Min', [],'MultiplexMode_Max', [])}}  showRawMsg=0  useSimFunc=0  sim_func_name=''  useStartVals=0  extendedId=0
      settings: SourceProductName=Raptor
  raptor_can_rxmsg2 : Raptor_lib/CAN/raptor_can_rxmsg  canDefinition=struct('dbcFile', 'SR26_CAN2.dbc','message', 'MM5_376','comment', '','signals', {{'MM5_ax','MM5_rollRate'}},'enabled', [ 1 1;],'scaled', [ 1 1;],'canBus', '''CAN2''','messageID', [ 376;],'idMask', [ 536870911;],'payloadMask', [],'payloadValue', [],'period', [ 0;],'mailbox', '''''','queueSize', [ 1;],'label', [ 0;],'ver', [ 2;],'showID', [ 0;],'showRaw', [ 0;],'showRawMsg', [ 0;],'useStartVals', [ 0;],'extendedId', [ 0;],'showAge', [ 1;],'useSimFunc', [ 0;],'sim_func_name', '''''','fill', [ 0;],'editID', [ 0;],'signalOrder', [ 1;],'signalAscDes', [ 1;],'msgLength', [ 8;])  canBus='CAN2'  mailbox=''  payloadMask=[]  payloadValue=[]  idMask=hex2dec('1FFFFFFF')  queueSize=1  showID=0  label=0  fill=0  id=376  showRaw=0  showAge=1  signalOrder=1  signalInfo={{struct('Name', 'MM5_ax','StartBit', [ 32;],'SignalSize', [ 16;],'ByteOrder', 'LittleEndian','ValueType', 'UNSIGNED','Class', 'uint16','Signed', [ 0;],'Factor', [ -0.0001274;],'Offset', [ 4.1746;],'Min', [ 0;],'Max', [ 0;],'Units', 'g','StartVal', [ 0;],'Comment', 'Acceleration X Axis','Multiplexed', [ 0;],'Multiplexor', [ 0;],'MultiplexMode_Min', [],'MultiplexMode_Max', []),struct('Name', 'MM5_rollRate','StartBit', [ 0;],'SignalSize', [ 16;],'ByteOrder', 'LittleEndian','ValueType', 'UNSIGNED','Class', 'uint16','Signed', [ 0;],'Factor', [ -0.005;],'Offset', [ 163.9;],'Min', [ 0;],'Max', [ 0;],'Units', 'deg/sec','StartVal', [ 0;],'Comment', 'Roll Rate','Multiplexed', [ 0;],'Multiplexor', [ 0;],'MultiplexMode_Min', [],'MultiplexMode_Max', [])}}  showRawMsg=0  useSimFunc=0  sim_func_name=''  useStartVals=0  extendedId=0
      settings: SourceProductName=Raptor
  raptor_can_rxmsg3 : Raptor_lib/CAN/raptor_can_rxmsg  canDefinition=struct('dbcFile', 'SR26_CAN2.dbc','message', 'MM52_450','comment', '','signals', {{'MM52_ay','MM52_yawRate'}},'enabled', [ 1 1;],'scaled', [ 1 1;],'canBus', '''CAN2''','messageID', [ 450;],'idMask', [ 536870911;],'payloadMask', [],'payloadValue', [],'period', [ 0;],'mailbox', '''''','queueSize', [ 1;],'label', [ 0;],'ver', [ 2;],'showID', [ 0;],'showRaw', [ 0;],'showRawMsg', [ 0;],'useStartVals', [ 0;],'extendedId', [ 0;],'showAge', [ 1;],'useSimFunc', [ 0;],'sim_func_name', '''''','fill', [ 0;],'editID', [ 0;],'signalOrder', [ 1;],'signalAscDes', [ 1;],'msgLength', [ 8;])  canBus='CAN2'  mailbox=''  payloadMask=[]  payloadValue=[]  idMask=hex2dec('1FFFFFFF')  queueSize=1  showID=0  label=0  fill=0  id=450  showRaw=0  showAge=1  signalOrder=1  signalInfo={{struct('Name', 'MM52_ay','StartBit', [ 32;],'SignalSize', [ 16;],'ByteOrder', 'LittleEndian','ValueType', 'UNSIGNED','Class', 'uint16','Signed', [ 0;],'Factor', [ 0.0001274;],'Offset', [ -4.1746;],'Min', [ 0;],'Max', [ 0;],'Units', 'g','StartVal', [ 0;],'Comment', 'Acceleration Y Axis','Multiplexed', [ 0;],'Multiplexor', [ 0;],'MultiplexMode_Min', [],'MultiplexMode_Max', []),struct('Name', 'MM52_yawRate','StartBit', [ 0;],'SignalSize', [ 16;],'ByteOrder', 'LittleEndian','ValueType', 'UNSIGNED','Class', 'uint16','Signed', [ 0;],'Factor', [ 0.005;],'Offset', [ -163.9;],'Min', [ 0;],'Max', [ 0;],'Units', 'deg/sec','StartVal', [ 0;],'Comment', 'Yaw Rate','Multiplexed', [ 0;],'Multiplexor', [ 0;],'MultiplexMode_Min', [],'MultiplexMode_Max', [])}}  showRawMsg=0  useSimFunc=0  sim_func_name=''  useStartVals=0  extendedId=0
      settings: SourceProductName=Raptor
  raptor_can_rxmsg4 : Raptor_lib/CAN/raptor_can_rxmsg  canDefinition=struct('dbcFile', 'SR26_CAN2.dbc','message', 'MM52_451','comment', '','signals', {{'MM52_ax','MM52_az','MM52_rollRate'}},'enabled', [ 1 1 1;],'scaled', [ 1 1 1;],'canBus', '''CAN2''','messageID', [ 451;],'idMask', [ 536870911;],'payloadMask', [],'payloadValue', [],'period', [ 0;],'mailbox', '''''','queueSize', [ 1;],'label', [ 0;],'ver', [ 2;],'showID', [ 0;],'showRaw', [ 0;],'showRawMsg', [ 0;],'useStartVals', [ 0;],'extendedId', [ 0;],'showAge', [ 1;],'useSimFunc', [ 0;],'sim_func_name', '''''','fill', [ 0;],'editID', [ 0;],'signalOrder', [ 1;],'signalAscDes', [ 1;],'msgLength', [ 8;])  canBus='CAN2'  mailbox=''  payloadMask=[]  payloadValue=[]  idMask=hex2dec('1FFFFFFF')  queueSize=1  showID=0  label=0  fill=0  id=451  showRaw=0  showAge=1  signalOrder=1  signalInfo={{struct('Name', 'MM52_az','StartBit', [ 32;],'SignalSize', [ 16;],'ByteOrder', 'LittleEndian','ValueType', 'UNSIGNED','Class', 'uint16','Signed', [ 0;],'Factor', [ -0.0001274;],'Offset', [ 4.1746;],'Min', [ 0;],'Max', [ 0;],'Units', 'g','StartVal', [ 0;],'Comment', 'Acceleration Z Axis','Multiplexed', [ 0;],'Multiplexor', [ 0;],'MultiplexMode_Min', [],'MultiplexMode_Max', []),struct('Name', 'MM52_ax','StartBit', [ 16;],'SignalSize', [ 16;],'ByteOrder', 'LittleEndian','ValueType', 'UNSIGNED','Class', 'uint16','Signed', [ 0;],'Factor', [ -0.0001274;],'Offset', [ 4.1746;],'Min', [ 0;],'Max', [ 0;],'Units', 'g','StartVal', [ 0;],'Comment', 'Acceleration X Axis','Multiplexed', [ 0;],'Multiplexor', [ 0;],'MultiplexMode_Min', [],'MultiplexMode_Max', []),struct('Name', 'MM52_rollRate','StartBit', [ 0;],'SignalSize', [ 16;],'ByteOrder', 'LittleEndian','ValueType', 'UNSIGNED','Class', 'uint16','Signed', [ 0;],'Factor', [ -0.005;],'Offset', [ 163.9;],'Min', [ 0;],'Max', [ 0;],'Units', 'deg/sec','StartVal', [ 0;],'Comment', 'Roll Rate','Multiplexed', [ 0;],'Multiplexor', [ 0;],'MultiplexMode_Min', [],'MultiplexMode_Max', [])}}  showRawMsg=0  useSimFunc=0  sim_func_name=''  useStartVals=0  extendedId=0
      settings: SourceProductName=Raptor
  raptor_can_rxmsg5 : Raptor_lib/CAN/raptor_can_rxmsg  canDefinition=struct('dbcFile', 'SR26_CAN2.dbc','message', 'MM5_380','comment', '','signals', {{'MM5_az'}},'enabled', [ 1;],'scaled', [ 1;],'canBus', '''CAN2''','messageID', [ 380;],'idMask', [ 536870911;],'payloadMask', [],'payloadValue', [],'period', [ 0;],'mailbox', '''''','queueSize', [ 1;],'label', [ 0;],'ver', [ 2;],'showID', [ 0;],'showRaw', [ 0;],'showRawMsg', [ 0;],'useStartVals', [ 0;],'extendedId', [ 0;],'showAge', [ 1;],'useSimFunc', [ 0;],'sim_func_name', '''''','fill', [ 0;],'editID', [ 0;],'signalOrder', [ 1;],'signalAscDes', [ 1;],'msgLength', [ 8;])  canBus='CAN2'  mailbox=''  payloadMask=[]  payloadValue=[]  idMask=hex2dec('1FFFFFFF')  queueSize=1  showID=0  label=0  fill=0  id=380  showRaw=0  showAge=1  signalOrder=1  signalInfo={{struct('Name', 'MM5_az','StartBit', [ 32;],'SignalSize', [ 16;],'ByteOrder', 'LittleEndian','ValueType', 'UNSIGNED','Class', 'uint16','Signed', [ 0;],'Factor', [ -0.0001274;],'Offset', [ 4.1746;],'Min', [ 0;],'Max', [ 0;],'Units', 'g','StartVal', [ 0;],'Comment', 'Acceleration Z Axis','Multiplexed', [ 0;],'Multiplexor', [ 0;],'MultiplexMode_Min', [],'MultiplexMode_Max', [])}}  showRawMsg=0  useSimFunc=0  sim_func_name=''  useStartVals=0  extendedId=0
      settings: SourceProductName=Raptor
  IO_CAN2_MM5_Bus : Outport
  wires:
  raptor_can_rxmsg4/4 -> Bus Creator4/4  "MM52_rollRate"
  Bus Creator5/1 -> Bus Creator/3  "IO_CAN2_380_Bus"
  raptor_can_rxmsg5/2 -> Bus Creator5/2  "MM5_az"
  raptor_can_rxmsg5/1 -> Bus Creator5/1  "Age"
  Bus Creator3/1 -> Bus Creator/4  "IO_CAN2_450_Bus"
  raptor_can_rxmsg3/2 -> Bus Creator3/2  "MM52_ay"
  raptor_can_rxmsg3/1 -> Bus Creator3/1  "Age"
  Bus Creator4/1 -> Bus Creator/5  "IO_CAN2_451Bus"
  raptor_can_rxmsg3/3 -> Bus Creator3/3  "MM52_yawRate"
  raptor_can_rxmsg4/2 -> Bus Creator4/2  "MM52_ax"
  raptor_can_rxmsg4/3 -> Bus Creator4/3  "MM52_az"
  raptor_can_rxmsg4/1 -> Bus Creator4/1  "Age"
  raptor_can_rxmsg2/1 -> Bus Creator2/1  "Age"
  raptor_can_rxmsg2/3 -> Bus Creator2/3  "MM5_rollRate"
  raptor_can_rxmsg2/2 -> Bus Creator2/2  "MM5_ax"
  raptor_can_rxmsg1/3 -> Bus Creator1/3  "MM5_yawRate"
  Bus Creator/1 -> IO_CAN2_MM5_Bus/1  "IO_CAN2_MM5_Bus"
  Bus Creator2/1 -> Bus Creator/2  "IO_CAN2_376_Bus"
  raptor_can_rxmsg1/1 -> Bus Creator1/1  "Age"
  raptor_can_rxmsg1/2 -> Bus Creator1/2  "MM5_ay"
  Bus Creator1/1 -> Bus Creator/1  "IO_CAN2_372_Bus"
